simulink model "scheme1mom"  (R2014a)
settings: Solver=ode45  StartTime=0.0  StopTime=0.4  MaxStep=0.001  MinStep=0.0001  RelTol=1e-3
settings Model: Creator=User  LastModifiedBy=Анастасия

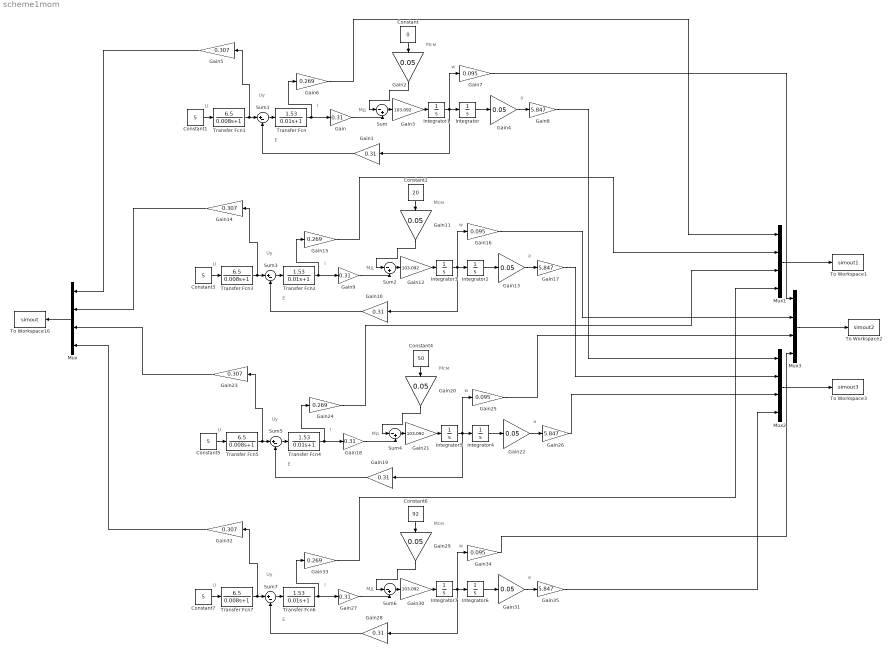
== system scheme1mom ==
  note: E
  note: a
  note: w
  note: Мд
  note: Mсм
  note: I
  note: Uy
  note: U
  note: E
  note: a
  note: w
  note: Мд
  note: Mсм
  note: I
  note: Uy
  note: U
  note: E
  note: a
  note: w
  note: Мд
  note: Mсм
  note: I
  note: Uy
  note: U
  note: E
  note: a
  note: w
  note: Мд
  note: Mсм
  note: I
  note: Uy
  note: U
  Constant : Constant  Value=0
  Constant{1,3,5,7} (4 alike) : Constant  Value=5
  Constant2 : Constant  Value=20
  Constant4 : Constant  Value=50
  Constant6 : Constant  Value=92
  Gain{,1,9..10,18..19,27..28} (8 alike) : Gain  Gain=0.31
  Gain{2,4,11,13,20,22,29,31} (8 alike) : Gain  Gain=0.05
  Gain{3,12,21,30} (4 alike) : Gain  Gain=103.092
  Gain{5,14,23,32} (4 alike) : Gain  Gain=0.307
  Gain{6,15,24,33} (4 alike) : Gain  Gain=0.269
  Gain{7,16,25,34} (4 alike) : Gain  Gain=0.095
  Gain{8,17,26,35} (4 alike) : Gain  Gain=5.847
  Integrator{,1..7} (8 alike) : Integrator
  Mux{,1..3} (4 alike) : Mux
  Sum{,2,4,6} (4 alike) : Sum  Inputs=|-+
  Sum{1,3,5,7} (4 alike) : Sum  Inputs=|+-
  To Workspace1 : ToWorkspace  VariableName=simout1  SaveFormat=Timeseries  SampleTime=-1
  To Workspace16 : ToWorkspace  VariableName=simout  SaveFormat=Timeseries  SampleTime=-1
  To Workspace2 : ToWorkspace  VariableName=simout2  SaveFormat=Timeseries  SampleTime=-1
  To Workspace3 : ToWorkspace  VariableName=simout3  SaveFormat=Timeseries  SampleTime=-1
  Transfer Fcn{,2,4,6} (4 alike) : TransferFcn  Numerator=[1.53]  Denominator=[0.01 1]
  Transfer Fcn{1,3,5,7} (4 alike) : TransferFcn  Numerator=[6.5]  Denominator=[0.008 1]
  wires:
  Constant1/1 -> Transfer Fcn1/1
  Transfer Fcn1/1 -> Gain5/1, Sum1/1
  Transfer Fcn/1 -> Gain6/1, Gain/1
  Gain/1 -> Sum/2
  Constant/1 -> Gain2/1
  Gain2/1 -> Sum/1
  Sum/1 -> Gain3/1
  Gain3/1 -> Integrator1/1
  Integrator1/1 -> Gain7/1, Gain1/1, Integrator/1
  Gain1/1 -> Sum1/2
  Sum1/1 -> Transfer Fcn/1
  Integrator/1 -> Gain4/1
  Gain4/1 -> Gain8/1
  Gain8/1 -> Mux2/1
  Gain7/1 -> Mux3/1
  Gain6/1 -> Mux1/1
  Gain5/1 -> Mux/1
  Constant3/1 -> Transfer Fcn3/1
  Transfer Fcn3/1 -> Gain14/1, Sum3/1
  Transfer Fcn2/1 -> Gain15/1, Gain9/1
  Gain9/1 -> Sum2/2
  Constant2/1 -> Gain11/1
  Gain11/1 -> Sum2/1
  Sum2/1 -> Gain12/1
  Gain12/1 -> Integrator3/1
  Integrator3/1 -> Gain16/1, Gain10/1, Integrator2/1
  Gain10/1 -> Sum3/2
  Sum3/1 -> Transfer Fcn2/1
  Integrator2/1 -> Gain13/1
  Gain13/1 -> Gain17/1
  Gain17/1 -> Mux2/2
  Gain16/1 -> Mux3/2
  Gain14/1 -> Mux/2
  Constant5/1 -> Transfer Fcn5/1
  Transfer Fcn5/1 -> Gain23/1, Sum5/1
  Transfer Fcn4/1 -> Gain24/1, Gain18/1
  Gain18/1 -> Sum4/2
  Constant4/1 -> Gain20/1
  Gain20/1 -> Sum4/1
  Sum4/1 -> Gain21/1
  Gain21/1 -> Integrator5/1
  Integrator5/1 -> Gain25/1, Gain19/1, Integrator4/1
  Gain19/1 -> Sum5/2
  Sum5/1 -> Transfer Fcn4/1
  Integrator4/1 -> Gain22/1
  Gain22/1 -> Gain26/1
  Gain26/1 -> Mux2/3
  Gain25/1 -> Mux3/3
  Gain23/1 -> Mux/3
  Constant7/1 -> Transfer Fcn7/1
  Transfer Fcn7/1 -> Gain32/1, Sum7/1
  Transfer Fcn6/1 -> Gain33/1, Gain27/1
  Gain27/1 -> Sum6/2
  Constant6/1 -> Gain29/1
  Gain29/1 -> Sum6/1
  Sum6/1 -> Gain30/1
  Gain30/1 -> Integrator7/1
  Integrator7/1 -> Gain34/1, Gain28/1, Integrator6/1
  Gain28/1 -> Sum7/2
  Sum7/1 -> Transfer Fcn6/1
  Integrator6/1 -> Gain31/1
  Gain31/1 -> Gain35/1
  Gain35/1 -> Mux2/4
  Gain34/1 -> Mux3/4
  Gain32/1 -> Mux/4
  Mux/1 -> To Workspace16/1
  Mux1/1 -> To Workspace1/1
  Gain15/1 -> Mux1/2
  Gain24/1 -> Mux1/3
  Gain33/1 -> Mux1/4
  Mux2/1 -> To Workspace3/1
  Mux3/1 -> To Workspace2/1
